simulink model "SNRvsBER"  (R2014a)
settings: Solver=ode45  StartTime=0.0  StopTime=100  RelTol=1e-3
undefined symbols (not defined in the file or in its folder): rsgenpoly
libraries: commutil2 x2, commblkcod2 x2, commdigbbndfm2 x2, commchan3 x1, commsink2 x1, commrandsrc2 x1
settings Model: Creator=HP  LastModifiedBy=HP

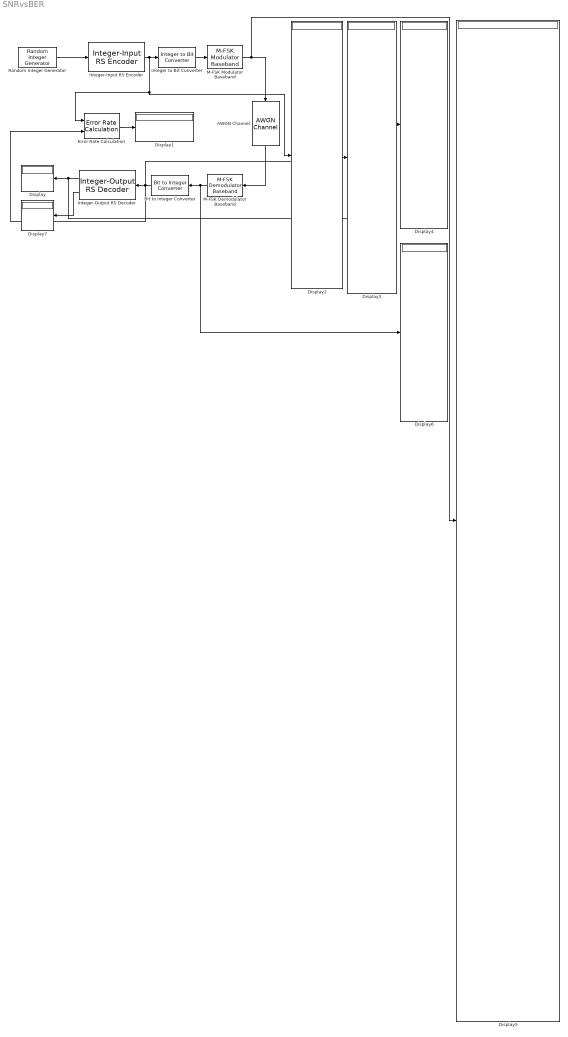
== system SNRvsBER ==
  AWGN Channel : commchan3/AWGN Channel  InputProcessing=Inherited (this choice will be removed - see release notes)  seed=67  noiseMode="Signal to noise ratio  (Eb/No)"  EbNodB=11.5  EsNodB=10  SNRdB=10  bitsPerSym=1  Ps=1  Tsym=1  variance=1
  Bit to Integer Converter : commutil2/Bit to Integer Converter  nbits=5  bitOrder=MSB first  signedOutputValues=Unsigned  outDtype=Inherit via internal rule  outDtypeSigned=Inherit via internal rule
  Display{,1..7} (8 alike) : Display
      Display1 settings: Format=long_e
      Display2 settings: Format=hex (Stored Integer)
      Display3 settings: Format=hex (Stored Integer)
      Display4 settings: Format=hex (Stored Integer)
      Display5 settings: Format=hex (Stored Integer)
      Display6 settings: Format=hex (Stored Integer)
  Error Rate Calculation : commsink2/Error Rate Calculation  N=0  st_delay=0  cp_mode=Entire frame  subframe=[]  PMode=Port  WsName=ErrorVec  RsMode2=off  stop=off  numErr=100  maxBits=1e6
  Integer to Bit Converter : commutil2/Integer to Bit Converter  nbits=5  signedInputValues=Unsigned  bitOrder=MSB first  outDtype=Inherit via internal rule
  Integer-Input RS Encoder : commblkcod2/Integer-Input RS Encoder  n=31  k=23  specPrimPoly=off  prPoly=[1 0 1 1]  specGenPoly=on  genPoly=rsgenpoly(31,23)  specPuncture=off  punctVec=[ones(2,1); zeros(2,1)]
  Integer-Output RS Decoder : commblkcod2/Integer-Output RS Decoder  n=31  k=23  specPrimPoly=off  prPoly=[1 0 1 1]  specGenPoly=on  genPoly=rsgenpoly(31,23)  specPuncture=off  punctVec=[ones(2,1); zeros(2,1)]  specErasurePort=off  showNumErr=on
  M-FSK Demodulator Baseband : commdigbbndfm2/M-FSK Demodulator Baseband  M=32  OutType=Bit  Dec=Gray  freqSep=6  numSamp=17  RateOptions=Enforce single-rate processing  outDataType=double
  M-FSK Modulator Baseband : commdigbbndfm2/M-FSK Modulator Baseband  M=32  InType=Bit  Enc=Gray  freqSep=6  phaseType=Continuous  numSamp=17  RateOptions=Enforce single-rate processing  outDataType=double
  Random Integer Generator : commrandsrc2/Random Integer Generator  mul=5  seed=37  Ts=1  frameBased=on  sampPerFrame=23  orient=off  outDataType=double
  wires:
  Random Integer Generator/1 -> Integer-Input RS Encoder/1
  Integer-Input RS Encoder/1 -> Display2/1, Error Rate Calculation/1, Integer to Bit Converter/1
  Integer to Bit Converter/1 -> M-FSK Modulator Baseband/1
  M-FSK Modulator Baseband/1 -> Display5/1, AWGN Channel/1
  AWGN Channel/1 -> M-FSK Demodulator Baseband/1
  M-FSK Demodulator Baseband/1 -> Display6/1, Bit to Integer Converter/1
  Bit to Integer Converter/1 -> Display3/1, Error Rate Calculation/2, Integer-Output RS Decoder/1
  Integer-Output RS Decoder/1 -> Display4/1, Display/1
  Error Rate Calculation/1 -> Display1/1
  Integer-Output RS Decoder/2 -> Display7/1
